simulink library "asbCubeSatEnvironmentLib"  (R2019a)
settings: Solver=VariableStepAuto  StartTime=0.0  StopTime=10.0  RelTol=1e-3
undefined symbols (not defined in the file): CubeSatTimeStep, initCond, km, s, vehicle
libraries: aerolibconvert2 x1, aerolibutil x1, aerolibgravity2 x1, aerolibcelestial x1
settings Model: Creator=The MathWorks, Inc.  LastModifiedBy=The MathWorks, Inc.
settings DataIOCC: ReturnWorkspaceOutputs=off
settings DebuggingCC: ArithmeticOperatorsInVariantConditions=warning

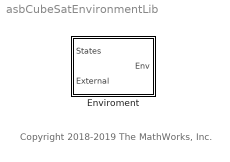
== system asbCubeSatEnvironmentLib ==
  note: Copyright 2018-2019 The MathWorks, Inc.
  Enviroment : Subsystem  RequirementInfo={} %GIDa_1ba82542_57ba_4b80_8f83_0a428ee4bc68

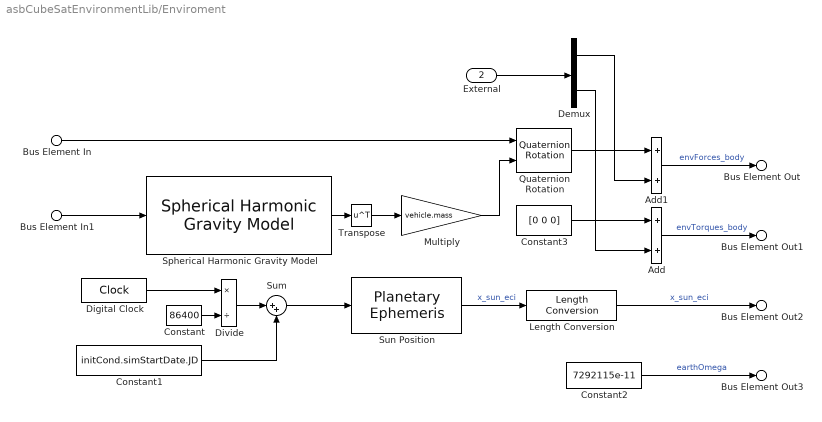
== system asbCubeSatEnvironmentLib/Enviroment ==
  Bus Element In : Inport  PortName=States  Element=q_ecef2b
  Bus Element In1 : Inport  PortName=States  Element=X_ecef
  External : Inport  RequirementInfo={} %GIDa_966e36cb_16b5_4872_900e_7ca1bd630c23  Port=2
  Add : Sum  RequirementInfo={} %GIDa_1e3b988f_8e92_4de4_9735_9df8703148df
  Add1 : Sum  RequirementInfo={} %GIDa_b8d2c483_28a5_4509_a823_93e900185cc4
  Constant : Constant  Value=86400
  Constant1 : Constant  RequirementInfo={} %GIDa_d3dce1ea_7a4c_4489_9b49_860fce94c68a  Value=initCond.simStartDate.JD
  Constant2 : Constant  RequirementInfo={} %GIDa_a027479b_4c7b_4f1d_b86b_1fc869131b24  Value=7292115e-11
  Constant3 : Constant  RequirementInfo={} %GIDa_08481c77_462d_49c1_8b19_5d7cc7c94401  Value=[0 0 0]
  Demux : Demux  RequirementInfo={} %GIDa_25e02362_af2f_4200_81e6_6d7271b48bfe  Outputs=2
  Digital Clock : DigitalClock  SampleTime=CubeSatTimeStep
  Divide : Product  Inputs=*/
  Length Conversion : aerolibconvert2/Length Conversion  IU=km  OU=m
  Multiply : Gain  Gain=vehicle.mass
  Quaternion Rotation : aerolibutil/Quaternion Rotation
  Spherical Harmonic Gravity Model : aerolibgravity2/Spherical Harmonic Gravity Model  RequirementInfo={} %GIDa_e6b23945_77d7_4eed_b23b_331bed44acc0  units=Metric (MKS)  degree=20  action=Warning  ptype=EGM2008  datafile='aerogmm2b.mat'
      settings: SourceProductName=Aerospace Blockset  SourceProductBaseCode=AE
  Sum : Sum  Inputs=|++
  Sun Position : aerolibcelestial/Planetary Ephemeris  kmflag=km,km/s  epochflag=Julian date  de=DE421  nCenter=Earth  nTarget=Sun  errorflag=Error  velflag=off
      settings: AttributesFormatString=Ephemeris Data Unavailable  SourceProductName=Aerospace Blockset  SourceProductBaseCode=AE
  Transpose : Math  RequirementInfo={} %GIDa_8c957334_dcef_4200_a34a_ed15bebfb21a  Operator=transpose  SaturateOnIntegerOverflow=on
  Bus Element Out : Outport  PortName=Env  Element=envForces_body
  Bus Element Out1 : Outport  PortName=Env  Element=envTorques_body
  Bus Element Out2 : Outport  PortName=Env  Element=x_sun_eci
  Bus Element Out3 : Outport  PortName=Env  Element=earthAngRate
  wires:
  Bus Element In1/1 -> Spherical Harmonic Gravity Model/1
  Bus Element In/1 -> Quaternion Rotation/1
  Constant3/1 -> Add/1
  Demux/1 -> Add1/2
  Quaternion Rotation/1 -> Add1/1
  Add1/1 -> Bus Element Out/1  "envForces_body"
  Add/1 -> Bus Element Out1/1  "envTorques_body"
  Demux/2 -> Add/2
  External/1 -> Demux/1
  Spherical Harmonic Gravity Model/1 -> Transpose/1
  Transpose/1 -> Multiply/1
  Sum/1 -> Sun Position/1
  Digital Clock/1 -> Divide/1
  Sun Position/1 -> Length Conversion/1  "x_sun_eci"
  Constant2/1 -> Bus Element Out3/1  "earthOmega"
  Length Conversion/1 -> Bus Element Out2/1  "x_sun_eci"
  Multiply/1 -> Quaternion Rotation/2
  Constant/1 -> Divide/2
  Divide/1 -> Sum/1
  Constant1/1 -> Sum/2
